simulink model "SORU2_Sekil11"  (R2018b)
settings: Solver=VariableStepAuto  StartTime=0.0  StopTime=200.0  RelTol=1e-3
settings Model: Creator=Fatih  LastModifiedBy=Fatih

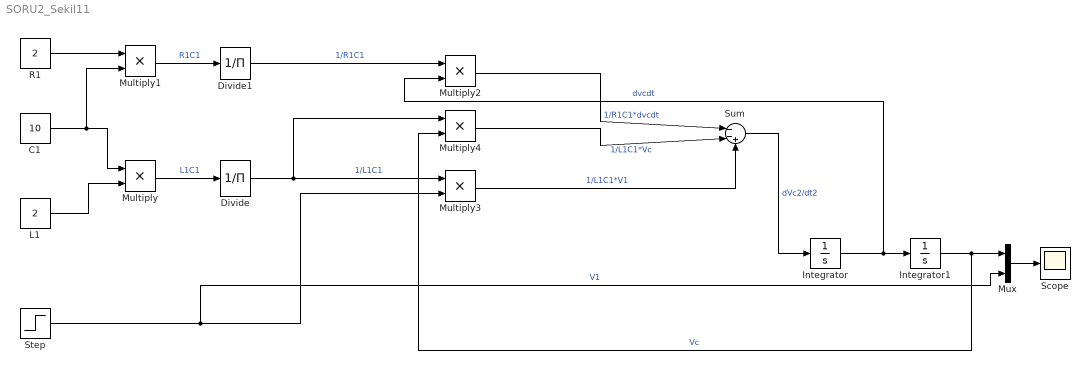
== system SORU2_Sekil11 ==
  "C1 " : Constant  Value=10
  Divide : Product  Inputs=/
  Divide1 : Product  Inputs=/
  Integrator : Integrator
  Integrator1 : Integrator
  "L1 " : Constant  Value=2
  Multiply{,1..4} (5 alike) : Product
  Mux : Mux  Inputs=2
  "R1 " : Constant  Value=2
  Scope : Scope
  Step : Step  SampleTime=0
  Sum : Sum  Inputs=|--+
  wires:
  "L1 "/1 -> Multiply/2
  "C1 "/1 -> Multiply1/2, Multiply/1
  Multiply/1 -> Divide/1  "L1C1"
  "R1 "/1 -> Multiply1/1
  Multiply1/1 -> Divide1/1  "R1C1"
  Divide1/1 -> Multiply2/1  "1/R1C1"
  Step/1 -> Multiply3/2, Mux/2  "V1"
  Divide/1 -> Multiply4/1, Multiply3/1  "1/L1C1"
  Integrator1/1 -> Multiply4/2, Mux/1  "Vc"
  Integrator/1 -> Multiply2/2, Integrator1/1  "dvcdt"
  Sum/1 -> Integrator/1  "dVc2/dt2"
  Multiply4/1 -> Sum/2  "1/L1C1*Vc"
  Multiply3/1 -> Sum/3  "1/L1C1*V1"
  Multiply2/1 -> Sum/1  "1/R1C1*dvcdt"
  Mux/1 -> Scope/1
